simulink library "ddm"  (R2021b)
settings: Solver=VariableStepAuto  StartTime=0.0  StopTime=10.0  RelTol=1e-3
undefined symbols (not defined in the file or in its folder): ENUM_ADASACCSTA_ERROR, ENUM_ADASACCSTA_OFF, ENUM_ADASACCSTA_STANDBY, ENUM_ADASISASTA_OFF, ENUM_ALLOWMOV_ALLOWREADY, ENUM_APS, ENUM_BRKSTA_ERROR, ENUM_BRKSTA_OFF, ENUM_BRKSTA_ON, ENUM_CHGPREACTERRSTA_OBCPRE, ENUM_DCDCFAULTSTA_ANYFAULTLV1, ENUM_DCDCFAULTSTA_ANYFAULTLV2, ENUM_DRIVETRAIN_AWD, ENUM_DRIVETRAIN_FWD, ENUM_DRIVETRAIN_RWD, ENUM_DRSEATSTA_INVALID, ENUM_EDUDRTSTA_NORMAL, ENUM_EPBSTA_APPLIED, ENUM_EPBSTA_RELEASED, ENUM_HVBATTREADYPRE_READY, ENUM_MCUWARN_LV0, ENUM_MCUWARN_LV1, ENUM_MCUWARN_LV2, ENUM_MCUWARN_LV3, ENUM_MCUWARN_NOERROR, ENUM_OBCFAULTSTA_ANYFAULT, ENUM_PAS_R2F2, ENUM_PDFAULT_BATTPDFAIL, ENUM_PDFAULT_DCDCDISABLE, ENUM_PDFAULT_MCUDISABLE, ENUM_PDFAULT_MCUDISCHRG, ENUM_POWERSTA_OFF, ENUM_POWERSTA_ON, ENUM_POWERSTA_READY, ENUM_POWERSTA_STANDBY, ENUM_PRESSINDI_LOW, ENUM_PUFAULT_BATTUPFAIL, ENUM_PUFAULT_DCDCENABLEFAIL, ENUM_PUFAULT_PRECHRGCHKFAIL, ENUM_PUFAULT_SAFETYCHKFAIL, ENUM_PUSTATE_COMPLETED, ENUM_PWRSTASW_OFF, ENUM_PWRSTASW_OFFA, ENUM_PWRSTASW_OFFCHVCHRG, ENUM_PWRSTASW_OFFCLVCHRG, ENUM_PWRSTASW_ON, ENUM_PWRSTASW_ONHVCHRG, ENUM_PWRSTASW_READY, ENUM_PWRSTASW_STANDBY, ENUM_RANGESTA_12IN, ENUM_RANGESTA_12OUT, ENUM_SHIFTCOMMAND_D, ENUM_SHIFTCOMMAND_N, ENUM_SHIFTCOMMAND_P, ENUM_SHIFTCOMMAND_R, ENUM_ZONEMALFUNLV_1ST, ENUM_ZONEMALFUNLV_2ND, ENUM_ZONEMALFUNLV_3RD, ENUM_ZONEMALFUNLV_4TH, ENUM_ZONESPDCTRLMODE_ACC ... (+832)
libraries: hcu_lib x738, $bdroot x26, simulink x7
(part 22 of 25)

== system ddm/DDM/DDM/VMC_DDM/FCM3/FCM3 Rolling Count Error  ==
  note: Fail Safe After Decision
  note: Release Condiction During Detection
  note: Diagnostics and Fault Handling
  note: Test Pass Criteria
  note: Release Condiction After Decision
  note: Test Detection Criteria
  note: Fail Safe During Detection
  task_time_s : Inport
  VDDM_FCM3RCErr_flg : Inport  Port=2
  No_CAN_BUS_OFF : Inport  Port=3
  VDDM_FCM3NoComCFS_flg : Inport  Port=4
  VPMM_PowerSta_enum : Inport  Port=5
  VINP_ADASACCSta_enum : Inport  Port=6
  VINP_ADASISASta_enum : Inport  Port=7
  DTC_clear_request : Inport  Port=8
  Constant : Constant  Value=ENUM_POWERSTA_OFF
  Constant1 : Constant  Value=ENUM_ADASACCSTA_OFF
  Constant{2,10,15,21,23} (5 alike) : Constant  Value=FALSE
  Constant{7,14,18,22} (4 alike) : Constant  Value=TRUE
  Constant16 : Constant  Value=ENUM_POWERSTA_STANDBY
  Constant17 : Constant  Value=ENUM_ADASISASTA_OFF
  Constant3 : Constant  Value=ENUM_ADASACCSTA_STANDBY
  Constant31 : Constant  Value=KDDM_FCM3RCErrDFSSW_flg
  Constant4 : Constant  Value=KDDM_FCM3RCErrCFSSW_flg
  Constant40 : Constant  Value=KDDM_FCM3RCErrDTC_cnt
  Constant41 : Constant  Value=KDDM_FCM3RCErrDetTO_ms
  Constant45 : Constant  Value=KDDM_FCM3RCErrPassSW_flg
  Constant46 : Constant  Value=KDDM_FCM3RCErrDetSW_flg
  Constant48 : Constant  Value=KDDM_FCM3RCErrDTC_cnt
  Constant5 : Constant  Value=ENUM_POWERSTA_OFF
  Constant6 : Constant  Value=KDDM_FCM3RCErrPassTO_ms
  Constant8 : Constant  Value=ENUM_POWERSTA_OFF
  Constant9 : Constant  Value=KDDM_FCM3RCErrPassTO_ms
  DTC_Couter : hcu_lib/Basic_Blocks/DTC_Couter
  DTC_Info : hcu_lib/Basic_Blocks/DTC_Info
  Data Type Conversion1 : DataTypeConversion  OutDataTypeStr=uint8
  Display : Display
  Display1 : Display
  Display2 : Display
  Equal : RelationalOperator  Operator=~=  OutDataTypeStr=boolean  RndMeth=Simplest
  Equal{1,8..11} (5 alike) : RelationalOperator  Operator===  OutDataTypeStr=boolean  RndMeth=Simplest
  Equal2 : RelationalOperator  Operator=~=  OutDataTypeStr=boolean  RndMeth=Simplest
  Equal3 : RelationalOperator  OutDataTypeStr=boolean  RndMeth=Simplest
  From6 : From  Commented=on  GotoTag=VDDM_EDriveSysErrVCUErr_flg
  Gain : Gain  Gain=XX2KXX
  Gain1 : Gain  Gain=KXX2XX
  Goto7 : Goto  Commented=on  GotoTag=VDDM_EDriveSysErrVCUErr_flg
  Logical Operator1 : Logic  Inputs=3  AllPortsSameDT=off  OutDataTypeStr=boolean
  Logical Operator10 : Logic  Operator=OR  AllPortsSameDT=off  OutDataTypeStr=boolean
  Logical Operator11 : Logic  Operator=OR  Inputs=3  AllPortsSameDT=off  OutDataTypeStr=boolean
  Logical Operator{4,12..13,15,18..19} (6 alike) : Logic  AllPortsSameDT=off  OutDataTypeStr=boolean
  Logical Operator16 : Logic  Operator=NOT  AllPortsSameDT=off  OutDataTypeStr=boolean
  Logical Operator2 : Logic  Inputs=3  AllPortsSameDT=off  OutDataTypeStr=boolean
  Logical Operator21 : Logic  Operator=OR  AllPortsSameDT=off  OutDataTypeStr=boolean
  Logical Operator3 : Logic  Operator=OR  AllPortsSameDT=off  OutDataTypeStr=boolean
  Logical Operator6 : Logic  Operator=NOT  AllPortsSameDT=off  OutDataTypeStr=boolean
  Relay : Relay  OnSwitchValue=ONE_INT  OffSwitchValue=ZERO_INT
  SR_Latch1 : hcu_lib/Basic_Blocks/SR_Latch
  SR_Latch3 : hcu_lib/Basic_Blocks/SR_Latch
  SR_Latch4 : hcu_lib/Basic_Blocks/SR_Latch
  Switch{,1..5} (6 alike) : Switch  Criteria=u2 ~= 0
  Terminator : Terminator
  Test Detection Criteria : hcu_lib/Basic_Blocks/Test Detection Criteria
  Timer1 : hcu_lib/Basic_Blocks/Timer
  Unit Delay1 : UnitDelay  SampleTime=-1  HasFrameUpgradeWarning=on
  VDDM_FCM3RCErrDFS_flg : Outport
  VDDM_FCM3RCErrCFS_flg : Outport  Port=2
  VDDM_FCM3RCErrDTC_raw32 : Outport  Port=3
  wires:
  VPMM_PowerSta_enum/1 -> [VPMM_PowerSta_enum]
  DTC_clear_request/1 -> [DTC_clear_request]
  No_CAN_BUS_OFF/1 -> [No_CAN_BUS_OFF]
  VINP_ADASACCSta_enum/1 -> [VINP_ADASACCSta_enum]
  VDDM_FCM3RCErr_flg/1 -> [VDDM_FCM3RCErr_flg]
  [VDDM_FCM3RCErrCFS_flg] -> VDDM_FCM3RCErrCFS_flg/1
  [VDDM_FCM3RCErrDFS_flg] -> VDDM_FCM3RCErrDFS_flg/1
  From6/1 -> Terminator/1
  Logical Operator6/1 -> Timer1/1
  Logical Operator21/1 -> SR_Latch3/2
  [VDDM_FCM3RCErrCFS_flg] -> Logical Operator21/2
  Constant22/1 -> Switch1/1
  [VDDM_xxx_flg] -> SR_Latch1/2
  [VDDM_FCM3RCErrCFS_flg] -> Switch/2
  Constant15/1 -> Switch4/3
  [VDDM_FCM3RCErrDTC_cnt] -> Relay/1
  Constant18/1 -> Switch/1
  Equal3/1 -> SR_Latch1/1
  Switch1/1 -> [VDDM_FCM3RCErrDFSRls_flg]
  Switch/1 -> Display1/1, Goto7/1
  Constant5/1 -> Equal2/2
  Constant2/1 -> Switch2/3
  Constant14/1 -> Switch4/1
  Logical Operator4/1 -> Switch3/2
  Constant7/1 -> Switch3/3
  Constant4/1 -> Logical Operator18/2
  [VDDM_FCM3RCErr_flg] -> Switch2/1
  [VDDM_FCM3RCErrCFSRls_flg] -> Logical Operator3/2
  Data Type Conversion1/1 -> [VDDM_FCM3RCErrDTC_cnt]
  Constant21/1 -> Switch/3
  [VDDM_FCM3RCErrCFSRls_flg] -> SR_Latch4/2
  Constant31/1 -> Logical Operator12/1
  [VDDM_FCM3RCErrPass_flg] -> Switch1/2
  Timer1/1 -> Equal3/1
  Constant23/1 -> Switch1/3
  [VDDM_FCM3RCErrDet_flg] -> Logical Operator19/1
  SR_Latch4/1 -> Logical Operator18/1
  Logical Operator2/1 -> Switch2/2
  Test Detection Criteria/1 -> [VDDM_FCM3RCErrDet_flg]
  [task_time_s] -> Test Detection Criteria/2
  Constant46/1 -> Logical Operator19/2
  Logical Operator12/1 -> [VDDM_FCM3RCErrDFS_flg]
  Constant41/1 -> Gain/1
  [VDDM_FCM3RCErrDFSRls_flg] -> Logical Operator21/1
  Switch4/1 -> Display2/1, [VDDM_FCM3RCErrCFSRls_flg]
  [VPMM_PowerSta_enum] -> Equal/1
  Switch3/1 -> Logical Operator6/1, Timer1/2
  Constant/1 -> Equal/2
  DTC_Couter/1 -> SR_Latch4/1
  Switch2/1 -> [VDDM_xxx_flg], Switch5/3
  [VDDM_FCM3RCErrPass_flg] -> Logical Operator3/1
  Constant45/1 -> Logical Operator15/2
  Logical Operator19/1 -> DTC_Couter/1
  [VDDM_FCM3RCErr_flg] -> Switch3/1
  [VPMM_PowerSta_enum] -> Equal2/1
  [No_CAN_BUS_OFF] -> Logical Operator4/1
  Constant48/1 -> DTC_Couter/3
  Equal2/1 -> Logical Operator4/2
  Logical Operator3/1 -> Logical Operator15/1
  Relay/1 -> SR_Latch3/1
  Logical Operator18/1 -> [VDDM_FCM3RCErrCFS_flg]
  Equal/1 -> Logical Operator2/3
  Gain/1 -> Test Detection Criteria/4
  SR_Latch1/1 -> Display/1, [VDDM_FCM3RCErrPass_flg]
  Constant6/1 -> Equal3/2
  Logical Operator15/1 -> DTC_Couter/2
  SR_Latch3/1 -> Logical Operator12/2
  Constant40/1 -> Test Detection Criteria/3
  DTC_Couter/2 -> Data Type Conversion1/1
  task_time_s/1 -> [task_time_s]  "task_time_s"
  Constant9/1 -> Timer1/4
  [VDDM_FCM3NoComCFS_flg] -> Logical Operator16/1
  Logical Operator16/1 -> Logical Operator2/2
  [No_CAN_BUS_OFF] -> Logical Operator2/1
  VDDM_FCM3NoComCFS_flg/1 -> [VDDM_FCM3NoComCFS_flg]
  Gain1/1 -> Timer1/3
  [task_time_s] -> Gain1/1
  [VINP_ADASISASta_enum] -> Equal1/1
  Equal1/1 -> Logical Operator1/3
  Equal9/1 -> Logical Operator10/2
  Constant3/1 -> Equal9/2
  Constant17/1 -> Equal1/2
  Equal11/1 -> Logical Operator13/2
  [VDDM_FCM3RCErrPass_flg] -> Logical Operator1/1
  Logical Operator13/1 -> Logical Operator11/2
  Constant1/1 -> Equal8/2
  [VPMM_PowerSta_enum] -> Equal11/1
  [VINP_ADASACCSta_enum] -> Equal9/1
  [VINP_ADASACCSta_enum] -> Equal8/1
  Logical Operator1/1 -> Logical Operator11/1
  Constant8/1 -> Equal10/2
  [DTC_clear_request] -> Logical Operator11/3
  Equal10/1 -> Logical Operator13/1
  Logical Operator10/1 -> Logical Operator1/2
  Equal8/1 -> Logical Operator10/1
  [VPMM_PowerSta_enum] -> Unit Delay1/1
  Unit Delay1/1 -> Equal10/1
  Constant16/1 -> Equal11/2
  Logical Operator11/1 -> Switch4/2
  VINP_ADASISASta_enum/1 -> [VINP_ADASISASta_enum]
  [DTC_clear_request] -> Switch5/2
  Constant10/1 -> Switch5/1
  Switch5/1 -> Test Detection Criteria/1
  [VDDM_FCM3RCErrDet_flg] -> DTC_Info/1
  [VDDM_FCM3RCErrPass_flg] -> DTC_Info/2
  [VDDM_FCM3RCErrCFS_flg] -> DTC_Info/3
  [DTC_clear_request] -> DTC_Info/4
  DTC_Info/1 -> VDDM_FCM3RCErrDTC_raw32/1  "VDDM_FCM3RCErrDTC_raw32"

== system ddm/DDM/DDM/VMC_DDM/FCM4/FCM4 Checksum Error  ==
  note: Fail Safe After Decision
  note: Release Condiction During Detection
  note: Diagnostics and Fault Handling
  note: Test Pass Criteria
  note: Release Condiction After Decision
  note: Test Detection Criteria
  note: Fail Safe During Detection
  task_time_s : Inport
  VDDM_FCM4CSErr_flg : Inport  Port=2
  No_CAN_BUS_OFF : Inport  Port=3
  VDDM_FCM4NoComCFS_flg : Inport  Port=4
  VPMM_PowerSta_enum : Inport  Port=5
  VINP_ADASACCSta_enum : Inport  Port=6
  DTC_clear_request : Inport  Port=7
  Constant : Constant  Value=ENUM_POWERSTA_OFF
  Constant{1..2,15,21,23} (5 alike) : Constant  Value=FALSE
  Constant10 : Constant  Value=ENUM_ADASACCSTA_OFF
  Constant11 : Constant  Value=ENUM_ADASACCSTA_STANDBY
  Constant12 : Constant  Value=ENUM_POWERSTA_OFF
  Constant13 : Constant  Value=ENUM_POWERSTA_STANDBY
  Constant{7,14,18,22} (4 alike) : Constant  Value=TRUE
  Constant31 : Constant  Value=KDDM_FCM4CSErrDFSSW_flg
  Constant4 : Constant  Value=KDDM_FCM4CSErrCFSSW_flg
  Constant40 : Constant  Value=KDDM_FCM4CSErrDTC_cnt
  Constant41 : Constant  Value=KDDM_FCM4CSErrDetTO_ms
  Constant45 : Constant  Value=KDDM_FCM4CSErrPassSW_flg
  Constant46 : Constant  Value=KDDM_FCM4CSErrDetSW_flg
  Constant48 : Constant  Value=KDDM_FCM4CSErrDTC_cnt
  Constant5 : Constant  Value=ENUM_POWERSTA_OFF
  Constant6 : Constant  Value=KDDM_FCM4CSErrPassTO_ms
  Constant9 : Constant  Value=KDDM_FCM4CSErrPassTO_ms
  DTC_Couter : hcu_lib/Basic_Blocks/DTC_Couter
  DTC_Info : hcu_lib/Basic_Blocks/DTC_Info
  Data Type Conversion1 : DataTypeConversion  OutDataTypeStr=uint8
  Display : Display
  Display1 : Display
  Display2 : Display
  Equal : RelationalOperator  Operator=~=  OutDataTypeStr=boolean  RndMeth=Simplest
  Equal2 : RelationalOperator  Operator=~=  OutDataTypeStr=boolean  RndMeth=Simplest
  Equal3 : RelationalOperator  OutDataTypeStr=boolean  RndMeth=Simplest
  Equal{4..7} (4 alike) : RelationalOperator  Operator===  OutDataTypeStr=boolean  RndMeth=Simplest
  From6 : From  Commented=on  GotoTag=VDDM_EDriveSysErrVCUErr_flg
  Gain : Gain  Gain=XX2KXX
  Gain1 : Gain  Gain=KXX2XX
  Goto7 : Goto  Commented=on  GotoTag=VDDM_EDriveSysErrVCUErr_flg
  Logical Operator{4..5,9,12,15,18..19} (7 alike) : Logic  AllPortsSameDT=off  OutDataTypeStr=boolean
  Logical Operator16 : Logic  Operator=NOT  AllPortsSameDT=off  OutDataTypeStr=boolean
  Logical Operator2 : Logic  Inputs=3  AllPortsSameDT=off  OutDataTypeStr=boolean
  Logical Operator21 : Logic  Operator=OR  AllPortsSameDT=off  OutDataTypeStr=boolean
  Logical Operator3 : Logic  Operator=OR  AllPortsSameDT=off  OutDataTypeStr=boolean
  Logical Operator6 : Logic  Operator=NOT  AllPortsSameDT=off  OutDataTypeStr=boolean
  Logical Operator7 : Logic  Operator=OR  AllPortsSameDT=off  OutDataTypeStr=boolean
  Logical Operator8 : Logic  Operator=OR  Inputs=3  AllPortsSameDT=off  OutDataTypeStr=boolean
  Relay : Relay  OnSwitchValue=ONE_INT  OffSwitchValue=ZERO_INT
  SR_Latch1 : hcu_lib/Basic_Blocks/SR_Latch
  SR_Latch3 : hcu_lib/Basic_Blocks/SR_Latch
  SR_Latch4 : hcu_lib/Basic_Blocks/SR_Latch
  Switch{,1..5} (6 alike) : Switch  Criteria=u2 ~= 0
  Terminator : Terminator
  Test Detection Criteria : hcu_lib/Basic_Blocks/Test Detection Criteria
  Timer1 : hcu_lib/Basic_Blocks/Timer
  Unit Delay2 : UnitDelay  SampleTime=-1  HasFrameUpgradeWarning=on
  VDDM_FCM4CSErrDFS_flg : Outport
  VDDM_FCM4CSErrCFS_flg : Outport  Port=2
  VDDM_FCM4CSErrDTC_raw32 : Outport  Port=3
  wires:
  VPMM_PowerSta_enum/1 -> [VPMM_PowerSta_enum]
  DTC_clear_request/1 -> [DTC_clear_request]
  No_CAN_BUS_OFF/1 -> [No_CAN_BUS_OFF]
  VINP_ADASACCSta_enum/1 -> [VINP_ADASACCSta_enum]
  VDDM_FCM4CSErr_flg/1 -> [VDDM_FCM4CSErr_flg]
  [VDDM_FCM4CSErrCFS_flg] -> VDDM_FCM4CSErrCFS_flg/1
  [VDDM_FCM4CSErrDFS_flg] -> VDDM_FCM4CSErrDFS_flg/1
  From6/1 -> Terminator/1
  Logical Operator6/1 -> Timer1/1
  Logical Operator21/1 -> SR_Latch3/2
  [VDDM_FCM4CSErrCFS_flg] -> Logical Operator21/2
  Constant22/1 -> Switch1/1
  [VDDM_xxx_flg] -> SR_Latch1/2
  [VDDM_FCM4CSErrCFS_flg] -> Switch/2
  [VINP_ADASACCSta_enum] -> Equal4/1
  [VPMM_PowerSta_enum] -> Unit Delay2/1
  Constant15/1 -> Switch4/3
  [VDDM_FCM4CSErrDTC_cnt] -> Relay/1
  Equal6/1 -> Logical Operator9/1
  Constant13/1 -> Equal7/2
  Constant18/1 -> Switch/1
  Equal3/1 -> SR_Latch1/1
  Switch1/1 -> [VDDM_FCM4CSErrDFSRls_flg]
  Switch/1 -> Display1/1, Goto7/1
  Constant5/1 -> Equal2/2
  [DTC_clear_request] -> Logical Operator8/3
  Unit Delay2/1 -> Equal6/1
  Constant12/1 -> Equal6/2
  Constant2/1 -> Switch2/3
  Logical Operator7/1 -> Logical Operator5/2
  Constant14/1 -> Switch4/1
  Logical Operator4/1 -> Switch3/2
  Equal4/1 -> Logical Operator7/1
  Equal5/1 -> Logical Operator7/2
  Constant7/1 -> Switch3/3
  Logical Operator5/1 -> Logical Operator8/1
  Constant4/1 -> Logical Operator18/2
  [VDDM_FCM4CSErr_flg] -> Switch2/1
  Equal7/1 -> Logical Operator9/2
  [VDDM_FCM4CSErrCFSRls_flg] -> Logical Operator3/2
  Data Type Conversion1/1 -> [VDDM_FCM4CSErrDTC_cnt]
  Constant21/1 -> Switch/3
  [VDDM_FCM4CSErrCFSRls_flg] -> SR_Latch4/2
  Constant31/1 -> Logical Operator12/1
  [VDDM_FCM4CSErrPass_flg] -> Switch1/2
  Timer1/1 -> Equal3/1
  Constant23/1 -> Switch1/3
  [VDDM_FCM4CSErrDet_flg] -> Logical Operator19/1
  SR_Latch4/1 -> Logical Operator18/1
  Logical Operator2/1 -> Switch2/2
  Test Detection Criteria/1 -> [VDDM_FCM4CSErrDet_flg]
  [task_time_s] -> Test Detection Criteria/2
  Constant46/1 -> Logical Operator19/2
  [VINP_ADASACCSta_enum] -> Equal5/1
  Logical Operator12/1 -> [VDDM_FCM4CSErrDFS_flg]
  Constant41/1 -> Gain/1
  [VDDM_FCM4CSErrDFSRls_flg] -> Logical Operator21/1
  Switch4/1 -> Display2/1, [VDDM_FCM4CSErrCFSRls_flg]
  Constant11/1 -> Equal5/2
  [VPMM_PowerSta_enum] -> Equal/1
  Switch3/1 -> Logical Operator6/1, Timer1/2
  Constant/1 -> Equal/2
  DTC_Couter/1 -> SR_Latch4/1
  Switch2/1 -> [VDDM_xxx_flg], Switch5/3
  [VDDM_FCM4CSErrPass_flg] -> Logical Operator3/1
  Constant45/1 -> Logical Operator15/2
  Logical Operator19/1 -> DTC_Couter/1
  [VDDM_FCM4CSErr_flg] -> Switch3/1
  [VPMM_PowerSta_enum] -> Equal2/1
  [VPMM_PowerSta_enum] -> Equal7/1
  Logical Operator8/1 -> Switch4/2
  Logical Operator9/1 -> Logical Operator8/2
  [No_CAN_BUS_OFF] -> Logical Operator4/1
  Constant10/1 -> Equal4/2
  Constant48/1 -> DTC_Couter/3
  Equal2/1 -> Logical Operator4/2
  [VDDM_FCM4CSErrPass_flg] -> Logical Operator5/1
  Logical Operator3/1 -> Logical Operator15/1
  Relay/1 -> SR_Latch3/1
  Logical Operator18/1 -> [VDDM_FCM4CSErrCFS_flg]
  Equal/1 -> Logical Operator2/3
  Gain/1 -> Test Detection Criteria/4
  SR_Latch1/1 -> Display/1, [VDDM_FCM4CSErrPass_flg]
  Constant6/1 -> Equal3/2
  Logical Operator15/1 -> DTC_Couter/2
  SR_Latch3/1 -> Logical Operator12/2
  Constant40/1 -> Test Detection Criteria/3
  DTC_Couter/2 -> Data Type Conversion1/1
  task_time_s/1 -> [task_time_s]  "task_time_s"
  Constant9/1 -> Timer1/4
  [VDDM_FCM4NoComCFS_flg] -> Logical Operator16/1
  Logical Operator16/1 -> Logical Operator2/2
  [No_CAN_BUS_OFF] -> Logical Operator2/1
  VDDM_FCM4NoComCFS_flg/1 -> [VDDM_FCM4NoComCFS_flg]
  [task_time_s] -> Gain1/1
  Gain1/1 -> Timer1/3
  [DTC_clear_request] -> Switch5/2
  Constant1/1 -> Switch5/1
  Switch5/1 -> Test Detection Criteria/1
  [VDDM_FCM4CSErrDet_flg] -> DTC_Info/1
  [VDDM_FCM4CSErrPass_flg] -> DTC_Info/2
  [VDDM_FCM4CSErrCFS_flg] -> DTC_Info/3
  [DTC_clear_request] -> DTC_Info/4
  DTC_Info/1 -> VDDM_FCM4CSErrDTC_raw32/1  "VDDM_FCM4CSErrDTC_raw32"

== system ddm/DDM/DDM/VMC_DDM/FCM4/FCM4 Lost Com ==
  note: Fail Safe After Decision
  note: Release Condiction During Detection
  note: Diagnostics and Fault Handling
  note: Test Pass Criteria
  note: Release Condiction After Decision
  note: Test Detection Criteria
  note: Fail Safe During Detection
  task_time_s : Inport
  VDDM_FCM4NoCom_flg : Inport  Port=2
  No_CAN_BUS_OFF : Inport  Port=3
  VPMM_PowerSta_enum : Inport  Port=4
  VINP_ADASACCSta_enum : Inport  Port=5
  DTC_clear_request : Inport  Port=6
  Constant : Constant  Value=ENUM_POWERSTA_OFF
  Constant{1..2,15,21,23} (5 alike) : Constant  Value=FALSE
  Constant10 : Constant  Value=ENUM_ADASACCSTA_OFF
  Constant11 : Constant  Value=ENUM_ADASACCSTA_STANDBY
  Constant12 : Constant  Value=ENUM_POWERSTA_OFF
  Constant13 : Constant  Value=ENUM_POWERSTA_STANDBY
  Constant{7,14,18,22} (4 alike) : Constant  Value=TRUE
  Constant31 : Constant  Value=KDDM_FCM4NoComDFSSW_flg
  Constant4 : Constant  Value=KDDM_FCM4NoComCFSSW_flg
  Constant40 : Constant  Value=KDDM_FCM4NoComDTC_cnt
  Constant41 : Constant  Value=KDDM_FCM4NoComDetTO_ms
  Constant45 : Constant  Value=KDDM_FCM4NoComPassSW_flg
  Constant46 : Constant  Value=KDDM_FCM4NoComDetSW_flg
  Constant48 : Constant  Value=KDDM_FCM4NoComDTC_cnt
  Constant5 : Constant  Value=ENUM_POWERSTA_OFF
  Constant6 : Constant  Value=KDDM_FCM4NoComPassTO_ms
  Constant9 : Constant  Value=KDDM_FCM4NoComPassTO_ms
  DTC_Couter : hcu_lib/Basic_Blocks/DTC_Couter
  DTC_Info : hcu_lib/Basic_Blocks/DTC_Info
  Data Type Conversion1 : DataTypeConversion  OutDataTypeStr=uint8
  Display : Display
  Display1 : Display
  Display2 : Display
  Equal : RelationalOperator  Operator=~=  OutDataTypeStr=boolean  RndMeth=Simplest
  Equal2 : RelationalOperator  Operator=~=  OutDataTypeStr=boolean  RndMeth=Simplest
  Equal3 : RelationalOperator  OutDataTypeStr=boolean  RndMeth=Simplest
  Equal{4..7} (4 alike) : RelationalOperator  Operator===  OutDataTypeStr=boolean  RndMeth=Simplest
  From6 : From  Commented=on  GotoTag=VDDM_EDriveSysErrVCUErr_flg
  Gain : Gain  Gain=XX2KXX
  Gain1 : Gain  Gain=KXX2XX
  Goto7 : Goto  Commented=on  GotoTag=VDDM_EDriveSysErrVCUErr_flg
  Logical Operator{2,4..5,9,12,15,18..19} (8 alike) : Logic  AllPortsSameDT=off  OutDataTypeStr=boolean
  Logical Operator21 : Logic  Operator=OR  AllPortsSameDT=off  OutDataTypeStr=boolean
  Logical Operator3 : Logic  Operator=OR  AllPortsSameDT=off  OutDataTypeStr=boolean
  Logical Operator6 : Logic  Operator=NOT  AllPortsSameDT=off  OutDataTypeStr=boolean
  Logical Operator7 : Logic  Operator=OR  AllPortsSameDT=off  OutDataTypeStr=boolean
  Logical Operator8 : Logic  Operator=OR  Inputs=3  AllPortsSameDT=off  OutDataTypeStr=boolean
  Relay : Relay  OnSwitchValue=ONE_INT  OffSwitchValue=ZERO_INT
  SR_Latch1 : hcu_lib/Basic_Blocks/SR_Latch
  SR_Latch3 : hcu_lib/Basic_Blocks/SR_Latch
  SR_Latch4 : hcu_lib/Basic_Blocks/SR_Latch
  Switch{,1..5} (6 alike) : Switch  Criteria=u2 ~= 0
  Terminator : Terminator
  Test Detection Criteria : hcu_lib/Basic_Blocks/Test Detection Criteria
  Timer1 : hcu_lib/Basic_Blocks/Timer
  Unit Delay2 : UnitDelay  SampleTime=-1  HasFrameUpgradeWarning=on
  VDDM_FCM4NoComDFS_flg : Outport
  VDDM_FCM4NoComCFS_flg : Outport  Port=2
  VDDM_FCM4NoComDTC_raw32 : Outport  Port=3
  wires:
  VPMM_PowerSta_enum/1 -> [VPMM_PowerSta_enum]
  DTC_clear_request/1 -> [DTC_clear_request]
  No_CAN_BUS_OFF/1 -> [No_CAN_BUS_OFF]
  VINP_ADASACCSta_enum/1 -> [VINP_ADASACCSta_enum]
  VDDM_FCM4NoCom_flg/1 -> [VDDM_FCM4NoCom_flg]
  [VDDM_FCM4NoComCFS_flg] -> VDDM_FCM4NoComCFS_flg/1
  [VDDM_FCM4NoComDFS_flg] -> VDDM_FCM4NoComDFS_flg/1
  From6/1 -> Terminator/1
  Logical Operator6/1 -> Timer1/1
  Logical Operator21/1 -> SR_Latch3/2
  [VDDM_FCM4NoComCFS_flg] -> Logical Operator21/2
  Constant22/1 -> Switch1/1
  [VDDM_xxx_flg] -> SR_Latch1/2
  [No_CAN_BUS_OFF] -> Logical Operator2/1
  [VDDM_FCM4NoComCFS_flg] -> Switch/2
  [VINP_ADASACCSta_enum] -> Equal4/1
  [VPMM_PowerSta_enum] -> Unit Delay2/1
  Constant15/1 -> Switch4/3
  [VDDM_FCM4NoComDTC_cnt] -> Relay/1
  [task_time_s] -> Gain1/1
  Equal6/1 -> Logical Operator9/1
  Constant13/1 -> Equal7/2
  Constant18/1 -> Switch/1
  Equal3/1 -> SR_Latch1/1
  Switch1/1 -> [VDDM_FCM4NoComDFSRls_flg]
  Switch/1 -> Display1/1, Goto7/1
  Constant5/1 -> Equal2/2
  [DTC_clear_request] -> Logical Operator8/3
  Unit Delay2/1 -> Equal6/1
  Constant12/1 -> Equal6/2
  Constant2/1 -> Switch2/3
  Logical Operator7/1 -> Logical Operator5/2
  Constant14/1 -> Switch4/1
  Logical Operator4/1 -> Switch3/2
  Equal4/1 -> Logical Operator7/1
  Equal5/1 -> Logical Operator7/2
  Constant7/1 -> Switch3/3
  Logical Operator5/1 -> Logical Operator8/1
  Constant4/1 -> Logical Operator18/2
  [VDDM_FCM4NoCom_flg] -> Switch2/1
  Equal7/1 -> Logical Operator9/2
  [VDDM_FCM4NoComCFSRls_flg] -> Logical Operator3/2
  Data Type Conversion1/1 -> [VDDM_FCM4NoComDTC_cnt]
  Constant21/1 -> Switch/3
  [VDDM_FCM4NoComCFSRls_flg] -> SR_Latch4/2
  Constant31/1 -> Logical Operator12/1
  [VDDM_FCM4NoComPass_flg] -> Switch1/2
  Timer1/1 -> Equal3/1
  Constant23/1 -> Switch1/3
  [VDDM_FCM4NoComDet_flg] -> Logical Operator19/1
  SR_Latch4/1 -> Logical Operator18/1
  Logical Operator2/1 -> Switch2/2
  Test Detection Criteria/1 -> [VDDM_FCM4NoComDet_flg]
  [task_time_s] -> Test Detection Criteria/2
  Constant46/1 -> Logical Operator19/2
  [VINP_ADASACCSta_enum] -> Equal5/1
  Logical Operator12/1 -> [VDDM_FCM4NoComDFS_flg]
  Constant41/1 -> Gain/1
  [VDDM_FCM4NoComDFSRls_flg] -> Logical Operator21/1
  Switch4/1 -> Display2/1, [VDDM_FCM4NoComCFSRls_flg]
  Constant11/1 -> Equal5/2
  [VPMM_PowerSta_enum] -> Equal/1
  Switch3/1 -> Logical Operator6/1, Timer1/2
  Constant/1 -> Equal/2
  DTC_Couter/1 -> SR_Latch4/1
  Switch2/1 -> [VDDM_xxx_flg], Switch5/3
  [VDDM_FCM4NoComPass_flg] -> Logical Operator3/1
  Constant45/1 -> Logical Operator15/2
  Logical Operator19/1 -> DTC_Couter/1
  [VDDM_FCM4NoCom_flg] -> Switch3/1
  [VPMM_PowerSta_enum] -> Equal2/1
  [VPMM_PowerSta_enum] -> Equal7/1
  Logical Operator8/1 -> Switch4/2
  Logical Operator9/1 -> Logical Operator8/2
  [No_CAN_BUS_OFF] -> Logical Operator4/1
  Constant10/1 -> Equal4/2
  Constant48/1 -> DTC_Couter/3
  Equal2/1 -> Logical Operator4/2
  [VDDM_FCM4NoComPass_flg] -> Logical Operator5/1
  Logical Operator3/1 -> Logical Operator15/1
  Relay/1 -> SR_Latch3/1
  Logical Operator18/1 -> [VDDM_FCM4NoComCFS_flg]
  Equal/1 -> Logical Operator2/2
  Gain/1 -> Test Detection Criteria/4
  SR_Latch1/1 -> Display/1, [VDDM_FCM4NoComPass_flg]
  Constant6/1 -> Equal3/2
  Logical Operator15/1 -> DTC_Couter/2
  SR_Latch3/1 -> Logical Operator12/2
  Constant40/1 -> Test Detection Criteria/3
  DTC_Couter/2 -> Data Type Conversion1/1
  task_time_s/1 -> [task_time_s]  "task_time_s"
  Gain1/1 -> Timer1/3
  Constant9/1 -> Timer1/4
  [DTC_clear_request] -> Switch5/2
  Constant1/1 -> Switch5/1
  Switch5/1 -> Test Detection Criteria/1
  [VDDM_FCM4NoComDet_flg] -> DTC_Info/1
  [VDDM_FCM4NoComPass_flg] -> DTC_Info/2
  [VDDM_FCM4NoComCFS_flg] -> DTC_Info/3
  [DTC_clear_request] -> DTC_Info/4
  DTC_Info/1 -> VDDM_FCM4NoComDTC_raw32/1  "VDDM_FCM4NoComDTC_raw32"

== system ddm/DDM/DDM/VMC_DDM/FCM4/FCM4 Rolling Count Error  ==
  note: Fail Safe After Decision
  note: Release Condiction During Detection
  note: Diagnostics and Fault Handling
  note: Test Pass Criteria
  note: Release Condiction After Decision
  note: Test Detection Criteria
  note: Fail Safe During Detection
  task_time_s : Inport
  VDDM_FCM4RCErr_flg : Inport  Port=2
  No_CAN_BUS_OFF : Inport  Port=3
  VDDM_FCM4NoComCFS_flg : Inport  Port=4
  VPMM_PowerSta_enum : Inport  Port=5
  VINP_ADASACCSta_enum : Inport  Port=6
  DTC_clear_request : Inport  Port=7
  Constant : Constant  Value=ENUM_POWERSTA_OFF
  Constant10 : Constant  Value=ENUM_ADASACCSTA_OFF
  Constant11 : Constant  Value=ENUM_ADASACCSTA_STANDBY
  Constant12 : Constant  Value=ENUM_POWERSTA_OFF
  Constant13 : Constant  Value=ENUM_POWERSTA_STANDBY
  Constant{7,14,18,22} (4 alike) : Constant  Value=TRUE
  Constant{2,15,21,23} (4 alike) : Constant  Value=FALSE
  Constant31 : Constant  Value=KDDM_FCM4RCErrDFSSW_flg
  Constant4 : Constant  Value=KDDM_FCM4RCErrCFSSW_flg
  Constant40 : Constant  Value=KDDM_FCM4RCErrDTC_cnt
  Constant41 : Constant  Value=KDDM_FCM4RCErrDetTO_ms
  Constant45 : Constant  Value=KDDM_FCM4RCErrPassSW_flg
  Constant46 : Constant  Value=KDDM_FCM4RCErrDetSW_flg
  Constant48 : Constant  Value=KDDM_FCM4RCErrDTC_cnt
  Constant5 : Constant  Value=ENUM_POWERSTA_OFF
  Constant6 : Constant  Value=KDDM_FCM4RCErrPassTO_ms
  Constant9 : Constant  Value=KDDM_FCM4RCErrPassTO_ms
  DTC_Couter : hcu_lib/Basic_Blocks/DTC_Couter
  Data Type Conversion1 : DataTypeConversion  OutDataTypeStr=uint8
  Display : Display
  Display1 : Display
  Display2 : Display
  Equal : RelationalOperator  Operator=~=  OutDataTypeStr=boolean  RndMeth=Simplest
  Equal2 : RelationalOperator  Operator=~=  OutDataTypeStr=boolean  RndMeth=Simplest
  Equal3 : RelationalOperator  OutDataTypeStr=boolean  RndMeth=Simplest
  Equal{4..7} (4 alike) : RelationalOperator  Operator===  OutDataTypeStr=boolean  RndMeth=Simplest
  From6 : From  Commented=on  GotoTag=VDDM_EDriveSysErrVCUErr_flg
  Gain : Gain  Gain=XX2KXX
  Gain1 : Gain  Gain=KXX2XX
  Goto7 : Goto  Commented=on  GotoTag=VDDM_EDriveSysErrVCUErr_flg
  Logical Operator{4..5,9,12,15,18..19} (7 alike) : Logic  AllPortsSameDT=off  OutDataTypeStr=boolean
  Logical Operator16 : Logic  Operator=NOT  AllPortsSameDT=off  OutDataTypeStr=boolean
  Logical Operator2 : Logic  Inputs=3  AllPortsSameDT=off  OutDataTypeStr=boolean
  Logical Operator21 : Logic  Operator=OR  AllPortsSameDT=off  OutDataTypeStr=boolean
  Logical Operator3 : Logic  Operator=OR  AllPortsSameDT=off  OutDataTypeStr=boolean
  Logical Operator6 : Logic  Operator=NOT  AllPortsSameDT=off  OutDataTypeStr=boolean
  Logical Operator7 : Logic  Operator=OR  AllPortsSameDT=off  OutDataTypeStr=boolean
  Logical Operator8 : Logic  Operator=OR  Inputs=3  AllPortsSameDT=off  OutDataTypeStr=boolean
  Relay : Relay  OnSwitchValue=ONE_INT  OffSwitchValue=ZERO_INT
  SR_Latch1 : Subsystem  mask(SR_Latch){}
      mask help: SR latch function.
  SR_Latch3 : hcu_lib/Basic_Blocks/SR_Latch
  SR_Latch4 : hcu_lib/Basic_Blocks/SR_Latch
  Switch{,1..4} (5 alike) : Switch  Criteria=u2 ~= 0
  Terminator : Terminator
  Test Detection Criteria : Subsystem
  Timer1 : Subsystem  mask(Timer){}
      mask help: Timer funcion.
  Unit Delay2 : UnitDelay  SampleTime=-1  HasFrameUpgradeWarning=on
  VDDM_FCM4RCErrDFS_flg : Outport
  VDDM_FCM4RCErrCFS_flg : Outport  Port=2
  wires:
  VPMM_PowerSta_enum/1 -> [VPMM_PowerSta_enum]
  DTC_clear_request/1 -> [DTC_clear_request]
  No_CAN_BUS_OFF/1 -> [No_CAN_BUS_OFF]
  VINP_ADASACCSta_enum/1 -> [VINP_ADASACCSta_enum]
  VDDM_FCM4RCErr_flg/1 -> [VDDM_FCM4RCErr_flg]
  [VDDM_FCM4RCErrCFS_flg] -> VDDM_FCM4RCErrCFS_flg/1
  [VDDM_FCM4RCErrDFS_flg] -> VDDM_FCM4RCErrDFS_flg/1
  From6/1 -> Terminator/1
  Logical Operator6/1 -> Timer1/1(trigger)
  Logical Operator21/1 -> SR_Latch3/2
  [VDDM_FCM4RCErrCFS_flg] -> Logical Operator21/2
  Constant22/1 -> Switch1/1
  [VDDM_FCM4RCErr_flg] -> SR_Latch1/2(reset)
  [VDDM_FCM4RCErrCFS_flg] -> Switch/2
  [VINP_ADASACCSta_enum] -> Equal4/1
  [VPMM_PowerSta_enum] -> Unit Delay2/1
  Constant15/1 -> Switch4/3
  [VDDM_FCM4RCErrDTC_cnt] -> Relay/1
  Equal6/1 -> Logical Operator9/1
  Constant13/1 -> Equal7/2
  Constant18/1 -> Switch/1
  Equal3/1 -> SR_Latch1/1(set)
  Switch1/1 -> [VDDM_FCM4RCErrDFSRls_flg]
  Switch/1 -> Display1/1, Goto7/1
  Constant5/1 -> Equal2/2
  [DTC_clear_request] -> Logical Operator8/3
  Unit Delay2/1 -> Equal6/1
  Constant12/1 -> Equal6/2
  Constant2/1 -> Switch2/3
  Logical Operator7/1 -> Logical Operator5/2
  Constant14/1 -> Switch4/1
  Logical Operator4/1 -> Switch3/2
  Equal4/1 -> Logical Operator7/1
  Equal5/1 -> Logical Operator7/2
  Constant7/1 -> Switch3/3
  Logical Operator5/1 -> Logical Operator8/1
  Constant4/1 -> Logical Operator18/2
  [VDDM_FCM4RCErr_flg] -> Switch2/1
  Equal7/1 -> Logical Operator9/2
  [VDDM_FCM4RCErrCFSRls_flg] -> Logical Operator3/2
  Data Type Conversion1/1 -> [VDDM_FCM4RCErrDTC_cnt]
  Constant21/1 -> Switch/3
  [VDDM_FCM4RCErrCFSRls_flg] -> SR_Latch4/2
  Constant31/1 -> Logical Operator12/1
  [VDDM_FCM4RCErrPass_flg] -> Switch1/2
  Timer1/1(time) -> Equal3/1
  Constant23/1 -> Switch1/3
  [VDDM_FCM4RCErrDet_flg] -> Logical Operator19/1
  SR_Latch4/1 -> Logical Operator18/1
  Logical Operator2/1 -> Switch2/2
  Test Detection Criteria/1(VDDM_xxxDet_flg) -> [VDDM_FCM4RCErrDet_flg]
  [task_time_s] -> Test Detection Criteria/2(Ts)
  Constant46/1 -> Logical Operator19/2
  [VINP_ADASACCSta_enum] -> Equal5/1
  Logical Operator12/1 -> [VDDM_FCM4RCErrDFS_flg]
  Constant41/1 -> Gain/1
  [VDDM_FCM4RCErrDFSRls_flg] -> Logical Operator21/1
  Switch4/1 -> Display2/1, [VDDM_FCM4RCErrCFSRls_flg]
  Constant11/1 -> Equal5/2
  [VPMM_PowerSta_enum] -> Equal/1
  Switch3/1 -> Logical Operator6/1, Timer1/2(reset)
  Constant/1 -> Equal/2
  DTC_Couter/1 -> SR_Latch4/1
  Switch2/1 -> Test Detection Criteria/1(trigger)
  [VDDM_FCM4RCErrPass_flg] -> Logical Operator3/1
  Constant45/1 -> Logical Operator15/2
  Logical Operator19/1 -> DTC_Couter/1
  [VDDM_FCM4RCErr_flg] -> Switch3/1
  [VPMM_PowerSta_enum] -> Equal2/1
  [VPMM_PowerSta_enum] -> Equal7/1
  Logical Operator8/1 -> Switch4/2
  Logical Operator9/1 -> Logical Operator8/2
  [No_CAN_BUS_OFF] -> Logical Operator4/1
  Constant10/1 -> Equal4/2
  Constant48/1 -> DTC_Couter/3
  Equal2/1 -> Logical Operator4/2
  [VDDM_FCM4RCErrPass_flg] -> Logical Operator5/1
  Logical Operator3/1 -> Logical Operator15/1
  Relay/1 -> SR_Latch3/1
  Logical Operator18/1 -> [VDDM_FCM4RCErrCFS_flg]
  Equal/1 -> Logical Operator2/3
  Gain/1 -> Test Detection Criteria/4(KDDM_xxxDetTO_s)
  SR_Latch1/1(latched) -> Display/1, [VDDM_FCM4RCErrPass_flg]
  Constant6/1 -> Equal3/2
  Logical Operator15/1 -> DTC_Couter/2
  SR_Latch3/1 -> Logical Operator12/2
  Constant40/1 -> Test Detection Criteria/3(KDDM_xxxDTC_cnt)
  DTC_Couter/2 -> Data Type Conversion1/1
  task_time_s/1 -> [task_time_s]  "task_time_s"
  Constant9/1 -> Timer1/4(max_time)
  [VDDM_FCM4NoComCFS_flg] -> Logical Operator16/1
  Logical Operator16/1 -> Logical Operator2/2
  [No_CAN_BUS_OFF] -> Logical Operator2/1
  VDDM_FCM4NoComCFS_flg/1 -> [VDDM_FCM4NoComCFS_flg]
  Gain1/1 -> Timer1/3(Ts)
  [task_time_s] -> Gain1/1

== system ddm/DDM/DDM/VMC_DDM/FCM5/FCM5 Checksum Error  ==
  note: Fail Safe After Decision
  note: Release Condiction During Detection
  note: Diagnostics and Fault Handling
  note: Test Pass Criteria
  note: Release Condiction After Decision
  note: Test Detection Criteria
  note: Fail Safe During Detection
  task_time_s : Inport
  VDDM_FCM5CSErr_flg : Inport  Port=2
  No_CAN_BUS_OFF : Inport  Port=3
  VDDM_FCM5NoComCFS_flg : Inport  Port=4
  VPMM_PowerSta_enum : Inport  Port=5
  VINP_ADASISASta_enum : Inport  Port=6
  DTC_clear_request : Inport  Port=7
  Constant : Constant  Value=ENUM_POWERSTA_OFF
  Constant{1..2,15,21,23} (5 alike) : Constant  Value=FALSE
  Constant{7,14,18,22} (4 alike) : Constant  Value=TRUE
  Constant16 : Constant  Value=ENUM_POWERSTA_STANDBY
  Constant17 : Constant  Value=ENUM_ADASISASTA_OFF
  Constant31 : Constant  Value=KDDM_FCM5CSErrDFSSW_flg
  Constant4 : Constant  Value=KDDM_FCM5CSErrCFSSW_flg
  Constant40 : Constant  Value=KDDM_FCM5CSErrDTC_cnt
  Constant41 : Constant  Value=KDDM_FCM5CSErrDetTO_ms
  Constant45 : Constant  Value=KDDM_FCM5CSErrPassSW_flg
  Constant46 : Constant  Value=KDDM_FCM5CSErrDetSW_flg
  Constant48 : Constant  Value=KDDM_FCM5CSErrDTC_cnt
  Constant5 : Constant  Value=ENUM_POWERSTA_OFF
  Constant6 : Constant  Value=KDDM_FCM5CSErrPassTO_ms
  Constant8 : Constant  Value=ENUM_POWERSTA_OFF
  Constant9 : Constant  Value=KDDM_FCM5CSErrPassTO_ms
  DTC_Couter : hcu_lib/Basic_Blocks/DTC_Couter
  DTC_Info : hcu_lib/Basic_Blocks/DTC_Info
  Data Type Conversion1 : DataTypeConversion  OutDataTypeStr=uint8
  Display : Display
  Display1 : Display
  Display2 : Display
  Equal : RelationalOperator  Operator=~=  OutDataTypeStr=boolean  RndMeth=Simplest
  Equal1 : RelationalOperator  Operator===  OutDataTypeStr=boolean  RndMeth=Simplest
  Equal10 : RelationalOperator  Operator===  OutDataTypeStr=boolean  RndMeth=Simplest
  Equal11 : RelationalOperator  Operator===  OutDataTypeStr=boolean  RndMeth=Simplest
  Equal2 : RelationalOperator  Operator=~=  OutDataTypeStr=boolean  RndMeth=Simplest
  Equal3 : RelationalOperator  OutDataTypeStr=boolean  RndMeth=Simplest
  From6 : From  Commented=on  GotoTag=VDDM_EDriveSysErrVCUErr_flg
  Gain : Gain  Gain=XX2KXX
  Gain1 : Gain  Gain=KXX2XX
  Goto7 : Goto  Commented=on  GotoTag=VDDM_EDriveSysErrVCUErr_flg
  Logical Operator{1,4,12..13,15,18..19} (7 alike) : Logic  AllPortsSameDT=off  OutDataTypeStr=boolean
  Logical Operator11 : Logic  Operator=OR  Inputs=3  AllPortsSameDT=off  OutDataTypeStr=boolean
  Logical Operator16 : Logic  Operator=NOT  AllPortsSameDT=off  OutDataTypeStr=boolean
  Logical Operator2 : Logic  Inputs=3  AllPortsSameDT=off  OutDataTypeStr=boolean
  Logical Operator21 : Logic  Operator=OR  AllPortsSameDT=off  OutDataTypeStr=boolean
  Logical Operator3 : Logic  Operator=OR  AllPortsSameDT=off  OutDataTypeStr=boolean
  Logical Operator6 : Logic  Operator=NOT  AllPortsSameDT=off  OutDataTypeStr=boolean
  Relay : Relay  OnSwitchValue=ONE_INT  OffSwitchValue=ZERO_INT
  SR_Latch1 : hcu_lib/Basic_Blocks/SR_Latch
  SR_Latch3 : hcu_lib/Basic_Blocks/SR_Latch
  SR_Latch4 : hcu_lib/Basic_Blocks/SR_Latch
  Switch{,1..5} (6 alike) : Switch  Criteria=u2 ~= 0
  Terminator : Terminator
  Test Detection Criteria : hcu_lib/Basic_Blocks/Test Detection Criteria
  Timer1 : hcu_lib/Basic_Blocks/Timer
  Unit Delay1 : UnitDelay  SampleTime=-1  HasFrameUpgradeWarning=on
  VDDM_FCM5CSErrDFS_flg : Outport
  VDDM_FCM5CSErrCFS_flg : Outport  Port=2
  VDDM_FCM5CSErrDTC_raw32 : Outport  Port=3
  wires:
  VPMM_PowerSta_enum/1 -> [VPMM_PowerSta_enum]
  DTC_clear_request/1 -> [DTC_clear_request]
  No_CAN_BUS_OFF/1 -> [No_CAN_BUS_OFF]
  VDDM_FCM5CSErr_flg/1 -> [VDDM_FCM5CSErr_flg]
  [VDDM_FCM5CSErrCFS_flg] -> VDDM_FCM5CSErrCFS_flg/1
  [VDDM_FCM5CSErrDFS_flg] -> VDDM_FCM5CSErrDFS_flg/1
  From6/1 -> Terminator/1
  Logical Operator6/1 -> Timer1/1
  Logical Operator21/1 -> SR_Latch3/2
  [VDDM_FCM5CSErrCFS_flg] -> Logical Operator21/2
  Constant22/1 -> Switch1/1
  [VDDM_xxx_flg] -> SR_Latch1/2
  [VDDM_FCM5CSErrCFS_flg] -> Switch/2
  Constant15/1 -> Switch4/3
  [VDDM_FCM5CSErrDTC_cnt] -> Relay/1
  Constant18/1 -> Switch/1
  Equal3/1 -> SR_Latch1/1
  Switch1/1 -> [VDDM_FCM5CSErrDFSRls_flg]
  Switch/1 -> Display1/1, Goto7/1
  Constant5/1 -> Equal2/2
  Constant2/1 -> Switch2/3
  Constant14/1 -> Switch4/1
  Logical Operator4/1 -> Switch3/2
  Constant7/1 -> Switch3/3
  Constant4/1 -> Logical Operator18/2
  [VDDM_FCM5CSErr_flg] -> Switch2/1
  [VDDM_FCM5CSErrCFSRls_flg] -> Logical Operator3/2
  Data Type Conversion1/1 -> [VDDM_FCM5CSErrDTC_cnt]
  Constant21/1 -> Switch/3
  [VDDM_FCM5CSErrCFSRls_flg] -> SR_Latch4/2
  Constant31/1 -> Logical Operator12/1
  [VDDM_FCM5CSErrPass_flg] -> Switch1/2
  Timer1/1 -> Equal3/1
  Constant23/1 -> Switch1/3
  [VDDM_FCM5CSErrDet_flg] -> Logical Operator19/1
  SR_Latch4/1 -> Logical Operator18/1
  Logical Operator2/1 -> Switch2/2
  Test Detection Criteria/1 -> [VDDM_FCM5CSErrDet_flg]
  [task_time_s] -> Test Detection Criteria/2
  Constant46/1 -> Logical Operator19/2
  Logical Operator12/1 -> [VDDM_FCM5CSErrDFS_flg]
  Constant41/1 -> Gain/1
  [VDDM_FCM5CSErrDFSRls_flg] -> Logical Operator21/1
  Switch4/1 -> Display2/1, [VDDM_FCM5CSErrCFSRls_flg]
  [VPMM_PowerSta_enum] -> Equal/1
  Switch3/1 -> Logical Operator6/1, Timer1/2
  Constant/1 -> Equal/2
  DTC_Couter/1 -> SR_Latch4/1
  Switch2/1 -> [VDDM_xxx_flg], Switch5/3
  [VDDM_FCM5CSErrPass_flg] -> Logical Operator3/1
  Constant45/1 -> Logical Operator15/2
  Logical Operator19/1 -> DTC_Couter/1
  [VDDM_FCM5CSErr_flg] -> Switch3/1
  [VPMM_PowerSta_enum] -> Equal2/1
  [No_CAN_BUS_OFF] -> Logical Operator4/1
  Constant48/1 -> DTC_Couter/3
  Equal2/1 -> Logical Operator4/2
  [VDDM_FCM5CSErrPass_flg] -> Logical Operator1/1
  Logical Operator3/1 -> Logical Operator15/1
  Relay/1 -> SR_Latch3/1
  Logical Operator18/1 -> [VDDM_FCM5CSErrCFS_flg]
  Equal/1 -> Logical Operator2/3
  Gain/1 -> Test Detection Criteria/4
  SR_Latch1/1 -> Display/1, [VDDM_FCM5CSErrPass_flg]
  Constant6/1 -> Equal3/2
  Logical Operator15/1 -> DTC_Couter/2
  SR_Latch3/1 -> Logical Operator12/2
  Constant40/1 -> Test Detection Criteria/3
  DTC_Couter/2 -> Data Type Conversion1/1
  task_time_s/1 -> [task_time_s]  "task_time_s"
  Constant9/1 -> Timer1/4
  [VDDM_FCM5NoComCFS_flg] -> Logical Operator16/1
  Logical Operator16/1 -> Logical Operator2/2
  [No_CAN_BUS_OFF] -> Logical Operator2/1
  VDDM_FCM5NoComCFS_flg/1 -> [VDDM_FCM5NoComCFS_flg]
  [task_time_s] -> Gain1/1
  Gain1/1 -> Timer1/3
  [VINP_ADASISASta_enum] -> Equal1/1
  Equal1/1 -> Logical Operator1/2
  Constant17/1 -> Equal1/2
  Equal11/1 -> Logical Operator13/2
  Logical Operator13/1 -> Logical Operator11/2
  [VPMM_PowerSta_enum] -> Equal11/1
  Logical Operator1/1 -> Logical Operator11/1
  Constant8/1 -> Equal10/2
  [DTC_clear_request] -> Logical Operator11/3
  Equal10/1 -> Logical Operator13/1
  [VPMM_PowerSta_enum] -> Unit Delay1/1
  Unit Delay1/1 -> Equal10/1
  Constant16/1 -> Equal11/2
  Logical Operator11/1 -> Switch4/2
  VINP_ADASISASta_enum/1 -> [VINP_ADASISASta_enum]
  Constant1/1 -> Switch5/1
  [DTC_clear_request] -> Switch5/2
  Switch5/1 -> Test Detection Criteria/1
  [VDDM_FCM5CSErrDet_flg] -> DTC_Info/1
  [VDDM_FCM5CSErrPass_flg] -> DTC_Info/2
  [VDDM_FCM5CSErrCFS_flg] -> DTC_Info/3
  [DTC_clear_request] -> DTC_Info/4
  DTC_Info/1 -> VDDM_FCM5CSErrDTC_raw32/1  "VDDM_FCM5CSErrDTC_raw32"

== system ddm/DDM/DDM/VMC_DDM/FCM5/FCM5 Lost Com ==
  note: Fail Safe After Decision
  note: Release Condiction During Detection
  note: Diagnostics and Fault Handling
  note: Test Pass Criteria
  note: Release Condiction After Decision
  note: Test Detection Criteria
  note: Fail Safe During Detection
  task_time_s : Inport
  VDDM_FCM5NoCom_flg : Inport  Port=2
  No_CAN_BUS_OFF : Inport  Port=3
  VPMM_PowerSta_enum : Inport  Port=4
  VINP_ADASISASta_enum : Inport  Port=5
  DTC_clear_request : Inport  Port=6
  Constant : Constant  Value=ENUM_POWERSTA_OFF
  Constant{1..2,15,21,23} (5 alike) : Constant  Value=FALSE
  Constant{7,14,18,22} (4 alike) : Constant  Value=TRUE
  Constant16 : Constant  Value=ENUM_POWERSTA_STANDBY
  Constant17 : Constant  Value=ENUM_ADASISASTA_OFF
  Constant31 : Constant  Value=KDDM_FCM5NoComDFSSW_flg
  Constant4 : Constant  Value=KDDM_FCM5NoComCFSSW_flg
  Constant40 : Constant  Value=KDDM_FCM5NoComDTC_cnt
  Constant41 : Constant  Value=KDDM_FCM5NoComDetTO_ms
  Constant45 : Constant  Value=KDDM_FCM5NoComPassSW_flg
  Constant46 : Constant  Value=KDDM_FCM5NoComDetSW_flg
  Constant48 : Constant  Value=KDDM_FCM5NoComDTC_cnt
  Constant5 : Constant  Value=ENUM_POWERSTA_OFF
  Constant6 : Constant  Value=KDDM_FCM5NoComPassTO_ms
  Constant8 : Constant  Value=ENUM_POWERSTA_OFF
  Constant9 : Constant  Value=KDDM_FCM5NoComPassTO_ms
  DTC_Couter : hcu_lib/Basic_Blocks/DTC_Couter
  DTC_Info : hcu_lib/Basic_Blocks/DTC_Info
  Data Type Conversion1 : DataTypeConversion  OutDataTypeStr=uint8
  Display : Display
  Display1 : Display
  Display2 : Display
  Equal : RelationalOperator  Operator=~=  OutDataTypeStr=boolean  RndMeth=Simplest
  Equal10 : RelationalOperator  Operator===  OutDataTypeStr=boolean  RndMeth=Simplest
  Equal11 : RelationalOperator  Operator===  OutDataTypeStr=boolean  RndMeth=Simplest
  Equal2 : RelationalOperator  Operator=~=  OutDataTypeStr=boolean  RndMeth=Simplest
  Equal3 : RelationalOperator  OutDataTypeStr=boolean  RndMeth=Simplest
  Equal8 : RelationalOperator  Operator===  OutDataTypeStr=boolean  RndMeth=Simplest
  From6 : From  Commented=on  GotoTag=VDDM_EDriveSysErrVCUErr_flg
  Gain : Gain  Gain=XX2KXX
  Gain1 : Gain  Gain=KXX2XX
  Goto7 : Goto  Commented=on  GotoTag=VDDM_EDriveSysErrVCUErr_flg
  Logical Operator{1..2,4,12..13,15,18..19} (8 alike) : Logic  AllPortsSameDT=off  OutDataTypeStr=boolean
  Logical Operator11 : Logic  Operator=OR  Inputs=3  AllPortsSameDT=off  OutDataTypeStr=boolean
  Logical Operator21 : Logic  Operator=OR  AllPortsSameDT=off  OutDataTypeStr=boolean
  Logical Operator3 : Logic  Operator=OR  AllPortsSameDT=off  OutDataTypeStr=boolean
  Logical Operator6 : Logic  Operator=NOT  AllPortsSameDT=off  OutDataTypeStr=boolean
  Relay : Relay  OnSwitchValue=ONE_INT  OffSwitchValue=ZERO_INT
  SR_Latch1 : hcu_lib/Basic_Blocks/SR_Latch
  SR_Latch3 : hcu_lib/Basic_Blocks/SR_Latch
  SR_Latch4 : hcu_lib/Basic_Blocks/SR_Latch
  Switch{,1..5} (6 alike) : Switch  Criteria=u2 ~= 0
  Terminator : Terminator
  Test Detection Criteria : hcu_lib/Basic_Blocks/Test Detection Criteria
  Timer1 : hcu_lib/Basic_Blocks/Timer
  Unit Delay1 : UnitDelay  SampleTime=-1  HasFrameUpgradeWarning=on
  VDDM_FCM5NoComDFS_flg : Outport
  VDDM_FCM5NoComCFS_flg : Outport  Port=2
  VDDM_FCM5NoComDTC_raw32 : Outport  Port=3
  wires:
  VPMM_PowerSta_enum/1 -> [VPMM_PowerSta_enum]
  DTC_clear_request/1 -> [DTC_clear_request]
  No_CAN_BUS_OFF/1 -> [No_CAN_BUS_OFF]
  VDDM_FCM5NoCom_flg/1 -> [VDDM_FCM5NoCom_flg]
  [VDDM_FCM5NoComCFS_flg] -> VDDM_FCM5NoComCFS_flg/1
  [VDDM_FCM5NoComDFS_flg] -> VDDM_FCM5NoComDFS_flg/1
  From6/1 -> Terminator/1
  Logical Operator6/1 -> Timer1/1
  Logical Operator21/1 -> SR_Latch3/2
  [VDDM_FCM5NoComCFS_flg] -> Logical Operator21/2
  Constant22/1 -> Switch1/1
  [VDDM_xxx_flg] -> SR_Latch1/2
  [No_CAN_BUS_OFF] -> Logical Operator2/1
  [VDDM_FCM5NoComCFS_flg] -> Switch/2
  Constant15/1 -> Switch4/3
  [VDDM_FCM5NoComDTC_cnt] -> Relay/1
  [task_time_s] -> Gain1/1
  Constant18/1 -> Switch/1
  Equal3/1 -> SR_Latch1/1
  Switch1/1 -> [VDDM_FCM5NoComDFSRls_flg]
  Switch/1 -> Display1/1, Goto7/1
  Constant5/1 -> Equal2/2
  Constant2/1 -> Switch2/3
  Constant14/1 -> Switch4/1
  Logical Operator4/1 -> Switch3/2
  Constant7/1 -> Switch3/3
  Constant4/1 -> Logical Operator18/2
  [VDDM_FCM5NoCom_flg] -> Switch2/1
  [VDDM_FCM5NoComCFSRls_flg] -> Logical Operator3/2
  Data Type Conversion1/1 -> [VDDM_FCM5NoComDTC_cnt]
  Constant21/1 -> Switch/3
  [VDDM_FCM5NoComCFSRls_flg] -> SR_Latch4/2
  Constant31/1 -> Logical Operator12/1
  [VDDM_FCM5NoComPass_flg] -> Switch1/2
  Timer1/1 -> Equal3/1
  Constant23/1 -> Switch1/3
  [VDDM_FCM5NoComDet_flg] -> Logical Operator19/1
  SR_Latch4/1 -> Logical Operator18/1
  Logical Operator2/1 -> Switch2/2
  Test Detection Criteria/1 -> [VDDM_FCM5NoComDet_flg]
  [task_time_s] -> Test Detection Criteria/2
  Constant46/1 -> Logical Operator19/2
  Logical Operator12/1 -> [VDDM_FCM5NoComDFS_flg]
  Constant41/1 -> Gain/1
  [VDDM_FCM5NoComDFSRls_flg] -> Logical Operator21/1
  Switch4/1 -> Display2/1, [VDDM_FCM5NoComCFSRls_flg]
  [VPMM_PowerSta_enum] -> Equal/1
  Switch3/1 -> Logical Operator6/1, Timer1/2
  Constant/1 -> Equal/2
  DTC_Couter/1 -> SR_Latch4/1
  Switch2/1 -> [VDDM_xxx_flg], Switch5/3
  [VDDM_FCM5NoComPass_flg] -> Logical Operator3/1
  Constant45/1 -> Logical Operator15/2
  Logical Operator19/1 -> DTC_Couter/1
  [VDDM_FCM5NoCom_flg] -> Switch3/1
  [VPMM_PowerSta_enum] -> Equal2/1
  Logical Operator11/1 -> Switch4/2
  [No_CAN_BUS_OFF] -> Logical Operator4/1
  Constant48/1 -> DTC_Couter/3
  Equal2/1 -> Logical Operator4/2
  [VDDM_FCM5NoComPass_flg] -> Logical Operator1/1
  Logical Operator3/1 -> Logical Operator15/1
  Relay/1 -> SR_Latch3/1
  Logical Operator18/1 -> [VDDM_FCM5NoComCFS_flg]
  Equal/1 -> Logical Operator2/2
  Gain/1 -> Test Detection Criteria/4
  SR_Latch1/1 -> Display/1, [VDDM_FCM5NoComPass_flg]
  Constant6/1 -> Equal3/2
  Logical Operator15/1 -> DTC_Couter/2
  SR_Latch3/1 -> Logical Operator12/2
  Constant40/1 -> Test Detection Criteria/3
  DTC_Couter/2 -> Data Type Conversion1/1
  task_time_s/1 -> [task_time_s]  "task_time_s"
  Constant9/1 -> Timer1/4
  Gain1/1 -> Timer1/3
  VINP_ADASISASta_enum/1 -> [VINP_ADASISASta_enum]
  [VPMM_PowerSta_enum] -> Unit Delay1/1
  Constant16/1 -> Equal11/2
  Unit Delay1/1 -> Equal10/1
  Logical Operator1/1 -> Logical Operator11/1
  Equal10/1 -> Logical Operator13/1
  [DTC_clear_request] -> Logical Operator11/3
  Constant8/1 -> Equal10/2
  Constant17/1 -> Equal8/2
  Equal11/1 -> Logical Operator13/2
  [VINP_ADASISASta_enum] -> Equal8/1
  Equal8/1 -> Logical Operator1/2
  [VPMM_PowerSta_enum] -> Equal11/1
  Logical Operator13/1 -> Logical Operator11/2
  Constant1/1 -> Switch5/1
  [DTC_clear_request] -> Switch5/2
  Switch5/1 -> Test Detection Criteria/1
  [VDDM_FCM5NoComDet_flg] -> DTC_Info/1
  [VDDM_FCM5NoComPass_flg] -> DTC_Info/2
  [VDDM_FCM5NoComCFS_flg] -> DTC_Info/3
  [DTC_clear_request] -> DTC_Info/4
  DTC_Info/1 -> VDDM_FCM5NoComDTC_raw32/1  "VDDM_FCM5NoComDTC_raw32"
